simulink model "controle_atitude"  (R2021b)
settings: Solver=ode45  StartTime=0.0  StopTime=1000  MaxStep=0.4  RelTol=1e-3
undefined symbols (not defined in the file): J, Jm, Jr, Ke, Km, Kt, L_a, R_a
libraries: aerolibutil x4, sharedutil x4, sharedtransform x3, slpidlib x1
settings Model: Creator=JRRL  LastModifiedBy=JRRL

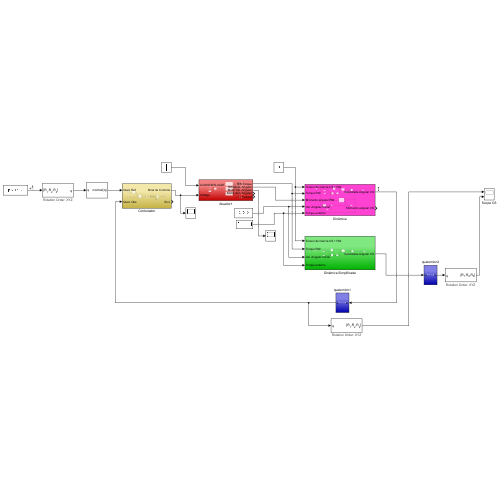
[thumbnail: Simulink's stored preview of the top-level diagram]
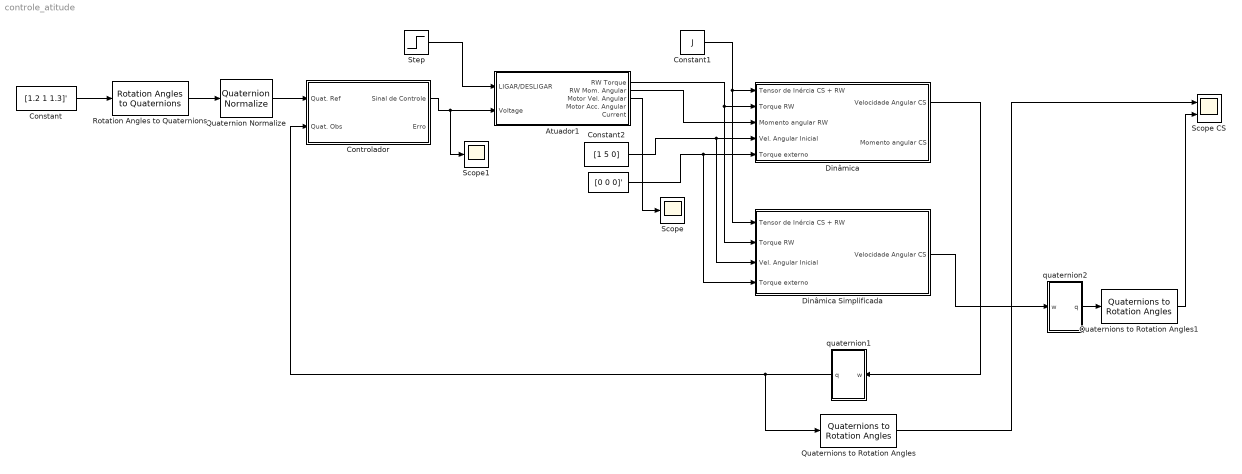
== system controle_atitude ==
  " " : Constant  Value=[0 0 0]'
  Atuador1 : Subsystem
  Constant : Constant  Value=[1.2 1 1.3]'
  Constant1 : Constant  Value=J
  Constant2 : Constant  Value=[1 5 0]
  Controlador : Subsystem
  Dinâmica : Subsystem
  Dinâmica Simplificada : Subsystem
  Quaternion Normalize : sharedutil/Quaternion Normalize  aMode=aMode
      settings: SourceProductBaseCode=AE,PW,DR,MT,UV,VE
  Quaternions to Rotation Angles : sharedtransform/Quaternions to Rotation Angles  rotationOrder=XYZ  aMode=aMode
      settings: SourceProductBaseCode=AE,PW,DR,MT,UV,VE
  Quaternions to Rotation Angles1 : sharedtransform/Quaternions to Rotation Angles  rotationOrder=XYZ  aMode=aMode
      settings: SourceProductBaseCode=AE,PW,DR,MT,UV,VE
  Rotation Angles to Quaternions : sharedtransform/Rotation Angles to Quaternions  rotationOrder=XYZ  aMode=aMode
      settings: SourceProductBaseCode=AE,PW,DR,MT,UV,VE
  Scope : Scope
  Scope CS : Scope  NumInputPorts=2
  Scope1 : Scope
  Step : Step  Time=100  Before=1  SampleTime=0
  quaternion1 : Subsystem
  quaternion2 : Subsystem
  wires:
  Constant1/1 -> Dinâmica Simplificada/1(Tensor de Inércia CS + RW), Dinâmica/1(Tensor de Inércia CS + RW)
  Dinâmica/1(Velocidade Angular CS) -> quaternion1/1(w)
  Constant/1 -> Rotation Angles to Quaternions/1
  Atuador1/1(RW Torque) -> Dinâmica Simplificada/2(Torque RW), Dinâmica/2(Torque RW)
  Constant2/1 -> Dinâmica Simplificada/3(Vel. Angular Inicial), Dinâmica/4(Vel. Angular Inicial)
  Controlador/1(Sinal de Controle) -> Scope1/1, Atuador1/2(Voltage)
  Rotation Angles to Quaternions/1 -> Quaternion Normalize/1
  Quaternion Normalize/1 -> Controlador/1(Quat. Ref)
  " "/1 -> Dinâmica Simplificada/4(Torque externo), Dinâmica/5(Torque externo)
  quaternion1/1(q) -> Quaternions to Rotation Angles/1, Controlador/2(Quat. Obs)
  Dinâmica Simplificada/1(Velocidade Angular CS) -> quaternion2/1(w)
  Quaternions to Rotation Angles/1 -> Scope CS/1
  quaternion2/1(q) -> Quaternions to Rotation Angles1/1
  Quaternions to Rotation Angles1/1 -> Scope CS/2
  Atuador1/2(RW Mom. Angular) -> Dinâmica/3(Momento angular RW)
  Step/1 -> Atuador1/1(LIGAR/DESLIGAR)
  Atuador1/3(Motor Vel. Angular) -> Scope/1

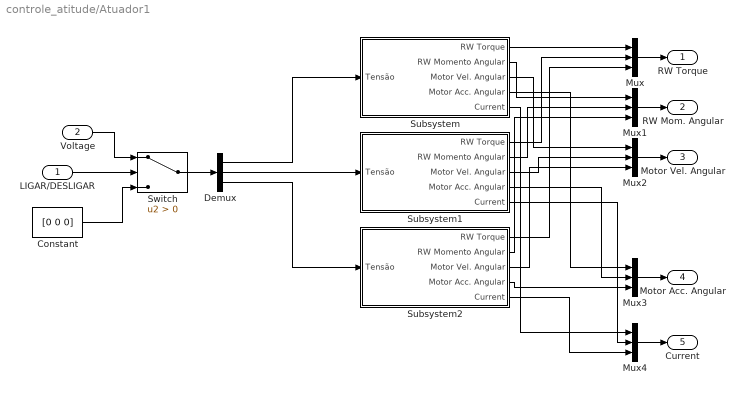
== system controle_atitude/Atuador1 ==
  LIGAR/DESLIGAR : Inport
  Voltage : Inport  Port=2
  Constant : Constant  Value=[0 0 0]
  Demux : Demux  Outputs=3
  Mux{,1..4} (5 alike) : Mux  Inputs=3
  Subsystem : Subsystem
  Subsystem1 : Subsystem
  Subsystem2 : Subsystem
  Switch : Switch  Criteria=u2 > Threshold
  RW Torque : Outport
  RW Mom. Angular : Outport  Port=2
  Motor Vel. Angular : Outport  Port=3
  Motor Acc. Angular : Outport  Port=4
  Current : Outport  Port=5
  wires:
  Switch/1 -> Demux/1
  Demux/2 -> Subsystem1/1(Tensão)
  Demux/3 -> Subsystem2/1(Tensão)
  Subsystem1/1(RW Torque) -> Mux/2
  Subsystem2/1(RW Torque) -> Mux/3
  Mux/1 -> RW Torque/1
  Mux1/1 -> RW Mom. Angular/1
  Mux2/1 -> Motor Vel. Angular/1
  Mux3/1 -> Motor Acc. Angular/1
  LIGAR/DESLIGAR/1 -> Switch/2
  Voltage/1 -> Switch/1
  Constant/1 -> Switch/3
  Demux/1 -> Subsystem/1(Tensão)
  Subsystem/1(RW Torque) -> Mux/1
  Subsystem/2(RW Momento Angular) -> Mux1/1
  Subsystem/3(Motor Vel. Angular) -> Mux2/1
  Subsystem/4(Motor Acc. Angular) -> Mux3/1
  Mux4/1 -> Current/1
  Subsystem/5(Current) -> Mux4/1
  Subsystem1/2(RW Momento Angular) -> Mux1/2
  Subsystem2/2(RW Momento Angular) -> Mux1/3
  Subsystem1/3(Motor Vel. Angular) -> Mux2/2
  Subsystem2/3(Motor Vel. Angular) -> Mux2/3
  Subsystem1/4(Motor Acc. Angular) -> Mux3/2
  Subsystem2/4(Motor Acc. Angular) -> Mux3/3
  Subsystem1/5(Current) -> Mux4/2
  Subsystem2/5(Current) -> Mux4/3

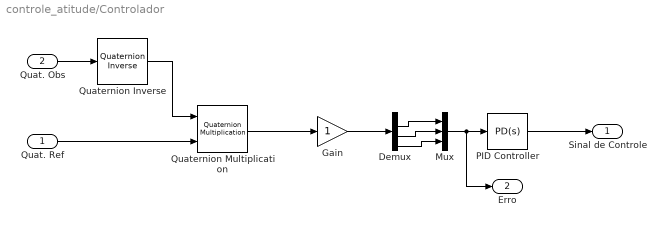
== system controle_atitude/Controlador ==
  Quat. Ref : Inport
  Quat. Obs : Inport  Port=2
  Demux : Demux
  Gain : Gain
  Mux : Mux  Inputs=3
  PID Controller : slpidlib/PID Controller  Controller=PD  Form=Parallel  TimeDomain=Continuous-time  UseExternalTs=off  SampleTime=-1  IntegratorMethod=Forward Euler  FilterMethod=Forward Euler  ControllerParametersSource=internal  P=6.919  I=0  D=65.829  UseFilter=on  N=100  TunerSelectOption=Transfer Function Based (PID Tuner App)  InitialConditionSource=internal  InitialConditionForIntegrator=0  InitialConditionForFilter=0  DifferentiatorICPrevScaledInput=0  ExternalReset=none  TrackingMode=off  Kt=1  LimitOutput=off  SatLimitsSource=internal  UpperSaturationLimit=inf  LowerSaturationLimit=-inf  LinearizeAsGain=on  AntiWindupMode=none  Kb=1  POutMin=[]  POutMax=[]  IOutMin=[]  IOutMax=[]  DOutMin=[]  DOutMax=[]  NOutMin=[]  NOutMax=[]  SumOutMin=[]  SumOutMax=[]  SaturationOutMin=[]  SaturationOutMax=[]  PParamMin=[]  PParamMax=[]  IParamMin=[]  IParamMax=[]  DParamMin=[]  DParamMax=[]  NParamMin=[]  NParamMax=[]  KbParamMin=[]  KbParamMax=[]  KtParamMin=[]  KtParamMax=[]  KbOutMin=[]  KbOutMax=[]  KtOutMin=[]  KtOutMax=[]  IntegratorOutMin=[]  IntegratorOutMax=[]  FilterOutMin=[]  FilterOutMax=[]  SumI1OutMin=[]  SumI1OutMax=[]  SumI2OutMin=[]  SumI2OutMax=[]  SumI3OutMin=[]  SumI3OutMax=[]  SumI4OutMin=[]  SumI4OutMax=[]  SumDOutMin=[]  SumDOutMax=[]  DifferentiatorOutMin=[]  DifferentiatorOutMax=[]  FilterDiffOutCoefMin=[]  FilterDiffOutCoefMax=[]  ReciprocalOutMin=[]  ReciprocalOutMax=[]  SumDenOutMin=[]  SumDenOutMax=[]  SumNumOutMin=[]  SumNumOutMax=[]  DivideOutMin=[]  DivideOutMax=[]  UdiffTsProdOutMin=[]  UdiffTsProdOutMax=[]  NTsProdOutMin=[]  NTsProdOutMax=[]  UintegralTsProdOutMin=[]  UintegralTsProdOutMax=[]  UngainTsProdOutMin=[]  UngainTsProdOutMax=[]  IntegratorContinuousStateAttributes=''  IntegratorStateMustResolveToSignalObject=off  IntegratorRTWStateStorageClass=Auto  FilterContinuousStateAttributes=''  FilterStateMustResolveToSignalObject=off  FilterRTWStateStorageClass=Auto  ParallelPVariant=InternalParameters  IdealPVariant=Disabled  IVariant=Disabled  DVariant=InternalParameters  IntegratorVariant=Disabled  SatVariant=Disabled  AWVariant=Disabled  PCopyVariant=Disabled  TRVariant=Disabled  FdbkBlocksVariant=Forward  IdealPFdbkVariant=Disabled  SatFdbkVariant=Disabled  DerivativeFilterVariant=ContFilter  NVariant=InternalParameters  NCopyVariant=Disabled  FilterICVariant=InternalICsFilter  IntegratorICVariant=Disabled  ExternalResetVariant=Disabled  TRSumVariant=Passthrough  SumFdbkVariant=Disabled  SumVariant=Sum_PD  TsampFilterVariant=InternalTs  TsampNgainVariant=Passthrough  TsampIntegralVariant=Disabled_SignalSpec  ExternalSaturationOutDataTypeStr=Inherit: Same as second input
  Quaternion Inverse : aerolibutil/Quaternion Inverse
  Quaternion Multiplication : aerolibutil/Quaternion Multiplication
  Sinal de Controle : Outport
  Erro : Outport  Port=2
  wires:
  Quat. Obs/1 -> Quaternion Inverse/1
  PID Controller/1 -> Sinal de Controle/1
  Quaternion Multiplication/1 -> Gain/1
  Demux/2 -> Mux/1
  Demux/3 -> Mux/2
  Demux/4 -> Mux/3
  Mux/1 -> Erro/1, PID Controller/1
  Quat. Ref/1 -> Quaternion Multiplication/2
  Quaternion Inverse/1 -> Quaternion Multiplication/1
  Gain/1 -> Demux/1

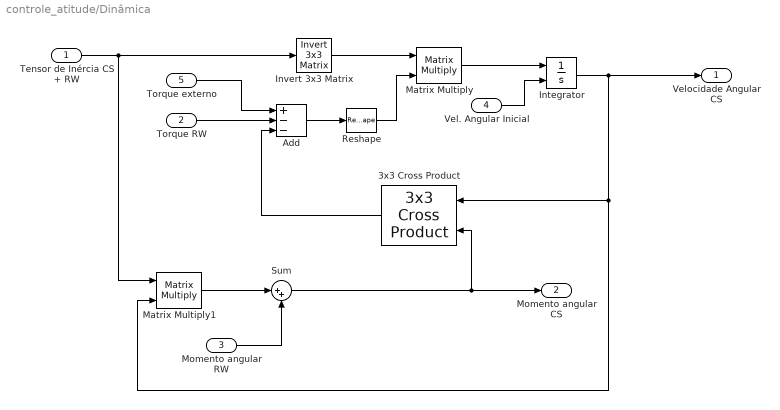
== system controle_atitude/Dinâmica ==
  Tensor de Inércia CS + RW : Inport
  Torque RW : Inport  Port=2
  Momento angular RW : Inport  Port=3
  Vel. Angular Inicial : Inport  Port=4
  Torque externo : Inport  Port=5
  3x3 Cross Product : sharedutil/3x3 Cross Product  aMode=aMode
      settings: SourceProductBaseCode=AE,PW,DR,MT,UV,VE
  Add : Sum  Inputs=+--
  Integrator : Integrator  InitialConditionSource=external
  Invert 3x3 Matrix : aerolibutil/Invert  3x3 Matrix
  Matrix Multiply : Product  Multiplication=Matrix(*)
  Matrix Multiply1 : Product  Multiplication=Matrix(*)
  Reshape : Reshape  OutputDimensionality=Column vector (2-D)
  Sum : Sum  Inputs=|++
  Velocidade Angular CS : Outport
  Momento angular CS : Outport  Port=2
  wires:
  Sum/1 -> Momento angular CS/1, 3x3 Cross Product/2
  3x3 Cross Product/1 -> Add/3
  Invert 3x3 Matrix/1 -> Matrix Multiply/1
  Integrator/1 -> Velocidade Angular CS/1, Matrix Multiply1/2, 3x3 Cross Product/1
  Matrix Multiply/1 -> Integrator/1
  Momento angular RW/1 -> Sum/2
  Torque RW/1 -> Add/2
  Tensor de Inércia CS + RW/1 -> Matrix Multiply1/1, Invert 3x3 Matrix/1
  Torque externo/1 -> Add/1
  Vel. Angular Inicial/1 -> Integrator/2
  Add/1 -> Reshape/1
  Matrix Multiply1/1 -> Sum/1
  Reshape/1 -> Matrix Multiply/2

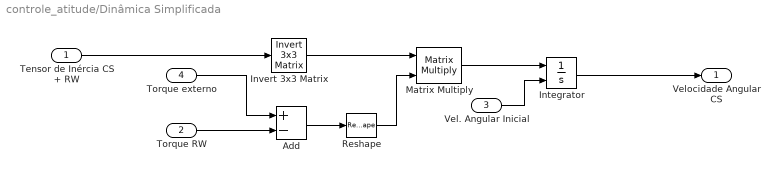
== system controle_atitude/Dinâmica Simplificada ==
  Tensor de Inércia CS + RW : Inport
  Torque RW : Inport  Port=2
  Vel. Angular Inicial : Inport  Port=3
  Torque externo : Inport  Port=4
  Add : Sum  Inputs=+-
  Integrator : Integrator  InitialConditionSource=external
  Invert 3x3 Matrix : aerolibutil/Invert  3x3 Matrix
  Matrix Multiply : Product  Multiplication=Matrix(*)
  Reshape : Reshape  OutputDimensionality=Column vector (2-D)
  Velocidade Angular CS : Outport
  wires:
  Add/1 -> Reshape/1
  Tensor de Inércia CS + RW/1 -> Invert 3x3 Matrix/1
  Torque RW/1 -> Add/2
  Vel. Angular Inicial/1 -> Integrator/2
  Reshape/1 -> Matrix Multiply/2
  Torque externo/1 -> Add/1
  Integrator/1 -> Velocidade Angular CS/1
  Invert 3x3 Matrix/1 -> Matrix Multiply/1
  Matrix Multiply/1 -> Integrator/1

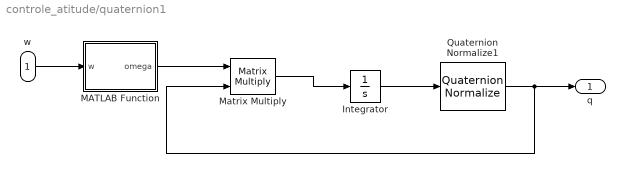
== system controle_atitude/quaternion1 ==
  w : Inport
  Integrator : Integrator  InitialCondition=[1 0 0 0]
  MATLAB Function : MATLAB Function  TreatAsAtomicUnit=on
  Matrix Multiply : Product  Multiplication=Matrix(*)
  Quaternion Normalize1 : sharedutil/Quaternion Normalize  aMode=aMode
      settings: SourceProductBaseCode=AE,PW,DR,MT,UV,VE
  q : Outport
  wires:
  w/1 -> MATLAB Function/1(w)
  MATLAB Function/1(omega) -> Matrix Multiply/1
  Quaternion Normalize1/1 -> q/1, Matrix Multiply/2
  Matrix Multiply/1 -> Integrator/1
  Integrator/1 -> Quaternion Normalize1/1

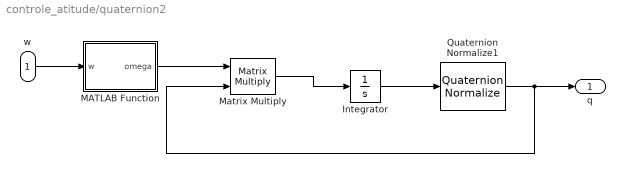
== system controle_atitude/quaternion2 ==
  w : Inport
  Integrator : Integrator  InitialCondition=[1 0 0 0]
  MATLAB Function : MATLAB Function  TreatAsAtomicUnit=on
  Matrix Multiply : Product  Multiplication=Matrix(*)
  Quaternion Normalize1 : sharedutil/Quaternion Normalize  aMode=aMode
      settings: SourceProductBaseCode=AE,PW,DR,MT,UV,VE
  q : Outport
  wires:
  w/1 -> MATLAB Function/1(w)
  MATLAB Function/1(omega) -> Matrix Multiply/1
  Quaternion Normalize1/1 -> q/1, Matrix Multiply/2
  Matrix Multiply/1 -> Integrator/1
  Integrator/1 -> Quaternion Normalize1/1

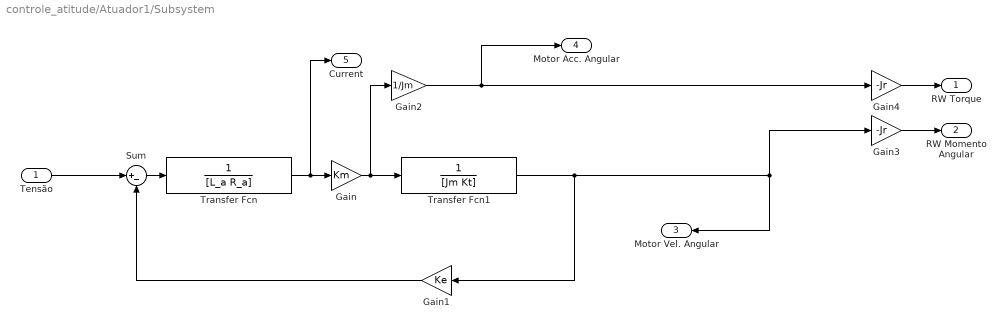
== system controle_atitude/Atuador1/Subsystem ==
  Tensão : Inport
  Gain : Gain  Gain=Km
  Gain1 : Gain  Gain=Ke
  Gain2 : Gain  Gain=1/Jm
  Gain3 : Gain  Gain=-Jr
  Gain4 : Gain  Gain=-Jr
  Sum : Sum  Inputs=|+-
  Transfer Fcn : TransferFcn  Denominator=[L_a R_a]
  Transfer Fcn1 : TransferFcn  Denominator=[Jm Kt]
  RW Torque : Outport
  RW Momento Angular : Outport  Port=2
  Motor Vel. Angular : Outport  Port=3
  Motor Acc. Angular : Outport  Port=4
  Current : Outport  Port=5
  wires:
  Gain/1 -> Transfer Fcn1/1, Gain2/1
  Transfer Fcn/1 -> Current/1, Gain/1
  Gain2/1 -> Gain4/1, Motor Acc. Angular/1
  Transfer Fcn1/1 -> Gain3/1, Motor Vel. Angular/1, Gain1/1
  Sum/1 -> Transfer Fcn/1
  Gain1/1 -> Sum/2
  Gain4/1 -> RW Torque/1
  Tensão/1 -> Sum/1
  Gain3/1 -> RW Momento Angular/1

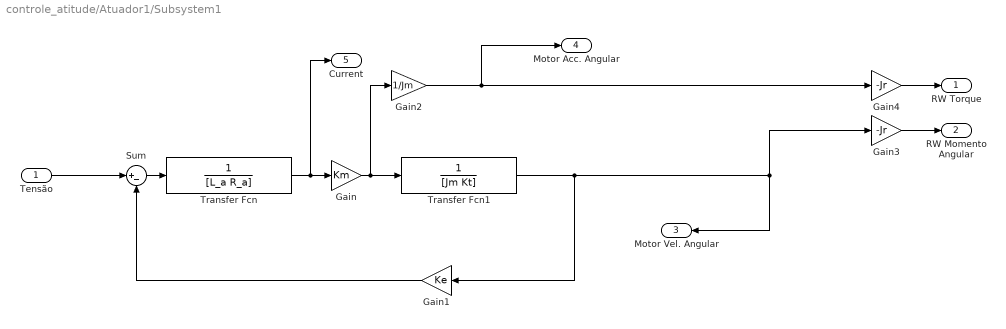
== system controle_atitude/Atuador1/Subsystem1 ==
  Tensão : Inport
  Gain : Gain  Gain=Km
  Gain1 : Gain  Gain=Ke
  Gain2 : Gain  Gain=1/Jm
  Gain3 : Gain  Gain=-Jr
  Gain4 : Gain  Gain=-Jr
  Sum : Sum  Inputs=|+-
  Transfer Fcn : TransferFcn  Denominator=[L_a R_a]
  Transfer Fcn1 : TransferFcn  Denominator=[Jm Kt]
  RW Torque : Outport
  RW Momento Angular : Outport  Port=2
  Motor Vel. Angular : Outport  Port=3
  Motor Acc. Angular : Outport  Port=4
  Current : Outport  Port=5
  wires:
  Gain/1 -> Transfer Fcn1/1, Gain2/1
  Transfer Fcn/1 -> Current/1, Gain/1
  Gain2/1 -> Gain4/1, Motor Acc. Angular/1
  Transfer Fcn1/1 -> Gain3/1, Motor Vel. Angular/1, Gain1/1
  Sum/1 -> Transfer Fcn/1
  Gain1/1 -> Sum/2
  Gain4/1 -> RW Torque/1
  Tensão/1 -> Sum/1
  Gain3/1 -> RW Momento Angular/1

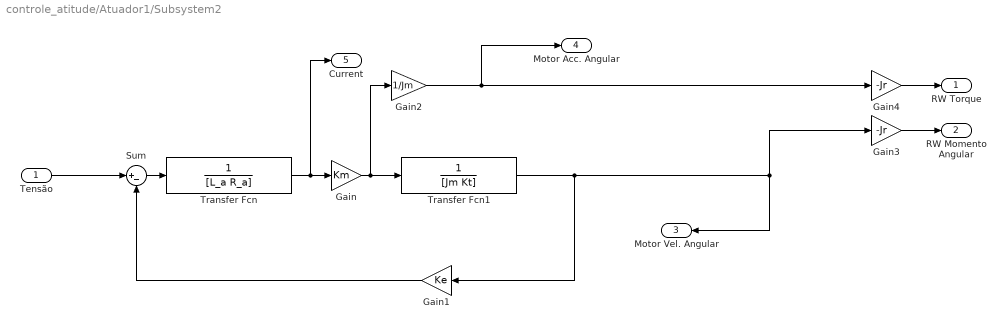
== system controle_atitude/Atuador1/Subsystem2 ==
  Tensão : Inport
  Gain : Gain  Gain=Km
  Gain1 : Gain  Gain=Ke
  Gain2 : Gain  Gain=1/Jm
  Gain3 : Gain  Gain=-Jr
  Gain4 : Gain  Gain=-Jr
  Sum : Sum  Inputs=|+-
  Transfer Fcn : TransferFcn  Denominator=[L_a R_a]
  Transfer Fcn1 : TransferFcn  Denominator=[Jm Kt]
  RW Torque : Outport
  RW Momento Angular : Outport  Port=2
  Motor Vel. Angular : Outport  Port=3
  Motor Acc. Angular : Outport  Port=4
  Current : Outport  Port=5
  wires:
  Gain/1 -> Transfer Fcn1/1, Gain2/1
  Transfer Fcn/1 -> Current/1, Gain/1
  Gain2/1 -> Gain4/1, Motor Acc. Angular/1
  Transfer Fcn1/1 -> Gain3/1, Motor Vel. Angular/1, Gain1/1
  Sum/1 -> Transfer Fcn/1
  Gain1/1 -> Sum/2
  Gain4/1 -> RW Torque/1
  Tensão/1 -> Sum/1
  Gain3/1 -> RW Momento Angular/1

== matlab function controle_atitude/quaternion1/MATLAB Function ==
  data: w input; omega output
function omega = fcn(w)
    wx = w(1);
    wy = w(2);
    wz = w(3);
    res = [0 -wx -wy -wz;wx 0 wz -wy;wy -wz 0 wx;wz wy -wx 0];
omega = res;

== matlab function controle_atitude/quaternion2/MATLAB Function ==
  data: w input; omega output
function omega = fcn(w)
    wx = w(1);
    wy = w(2);
    wz = w(3);
    res = [0 -wx -wy -wz;wx 0 wz -wy;wy -wz 0 wx;wz wy -wx 0];
omega = res;
